simulink model "mysvm_svc"  (R2017b)
settings: Solver=ode45  StartTime=0.0  StopTime=0.02  RelTol=1e-3  EnableMultiTasking=on
values from neighbouring files (symbols this model uses):
  N = nlcinput(4) - 1    [MLNLC_m.m]    (also in MLPDPWM_m.m = pdpwminput(4) - 1; MLSVC_m.m = svcinput(4) - 1; MLSVM_m_HD.m = svminput(5) - 1; PlotSpaceVector.m = block.DialogPrm(1).Data - 1)
undefined symbols (not defined in the file or in its folder): m
libraries: powerlib x5, powerlib_meascontrol x5
settings Model: Creator=吴鸿达  LastModifiedBy=AdamWu
settings DataIOCC: LimitDataPoints=on  SaveFormat=Array
settings OptimizationCC: LifeSpan=inf
settings DebuggingCC: SolverPrmCheckMsg=warning  SFUnexpectedBacktrackingDiag=warning  SFNoUnconditionalDefaultTransitionDiag=warning  SFExecutionAtInitializationDiag=none
settings HardwareCC: ProdBitPerPointer=32  ProdBitPerSizeT=32  ProdBitPerPtrDiffT=32  ProdLargestAtomicFloat=None  ProdIntDivRoundTo=Undefined  ProdEndianess=Unspecified  ProdWordSize=32  ProdHWDeviceType=32-bit Generic
settings ModelReferenceCC: PropagateSignalLabelsOutOfModel=off
settings CodeAppCC: StateflowObjectComments=on
settings GRTTargetCC: TargetLangStandard=C89/C90 (ANSI)  GeneratePreprocessorConditionals=Disable all
settings ConfigComp: CovMetricSettings=dw  CovHtmlReporting=on  CovSaveCumulativeToWorkspaceVar=on  CovSaveSingleToWorkspaceVar=on  CovExternalEMLEnable=off  CovSFcnEnable=off
settings SimscapeCC: SimscapeNormalizeSystem=off

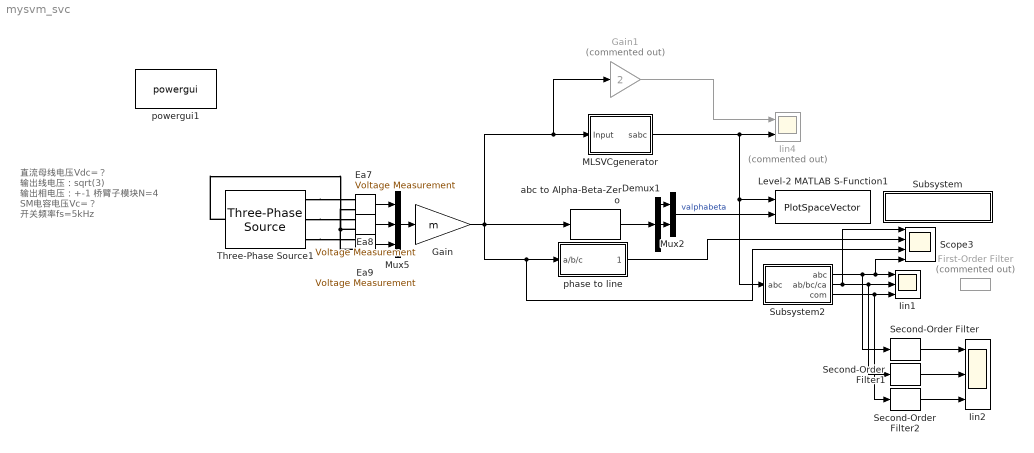
== system mysvm_svc ==
  note: 直流母线电压Vdc=？
      |
      | 输出线电压：sqrt(3)
      | 输出相电压：+-1
      | 桥臂子模块N=4
      | SM电容电压Vc=？
      | 开关频率fs=5kHz
  Demux1 : Demux  Outputs=3
  Ea7 : powerlib/Measurements/Voltage Measurement  PhasorSimulation=off  OutputType=Complex  PSBequivalent=0
  Ea8 : powerlib/Measurements/Voltage Measurement  PhasorSimulation=off  OutputType=Complex  PSBequivalent=0
  Ea9 : powerlib/Measurements/Voltage Measurement  PhasorSimulation=off  OutputType=Complex  PSBequivalent=0
  First-Order Filter : powerlib_meascontrol/Filters/First-Order Filter  Commented=on  FilterType=Lowpass  Tc=3.7e-4  Ts=0  Initialize=on  Vac_Init=[0, 0, 50]  Vdc_Init=0  PlotResponse=off  FreqRange="[0,  2000,  1]"
      settings: SourceProductName=Simscape Power Systems
  Gain : Gain  Gain=m
  Gain1 : Gain  Commented=on  Gain=2
  Iin1 : Scope  NumInputPorts=3
  Iin2 : Scope  NumInputPorts=3
  Iin4 : Scope  Commented=on  NumInputPorts=2
  Level-2 MATLAB S-Function1 : M-S-Function  FunctionName=PlotSpaceVector  Parameters=level, vdc, rate, normalized, plot, hexagon, sw, disabled  mask{disabled=off, level=N, rate=100, vdc=2/50, normalized=on, plot=5, hexagon=off, sw=off}
      mask prompts: disabled "Disable Plot"; level "Voltage Level"; rate "Plot Rate"; vdc "DC Link Voltage"; plot "Plot Number"; sw "Show Switching"
  MLSVCgenerator : Subsystem  mask{level=N, method=15. Zero Common Voltage}
      mask prompts: level "Voltage Level"
      mask TypeOptions method: 1. Conventional (x-y) | 2. x-y (iterative) | 3. H-D | 4. H-D (iterative) | 5. B-J-120 | 6. B-J-120 (iterative) | 7. B-J-60 | 8. B-J-60 (iterative) | 9. A-B-C | 10. A-B-C (iterative) | 11. Six-Axes | 12. Six-Axes (iterative) | 13. Shifted H-D | 14. Shifted B-J-60 | 15. Zero Common Voltage
  Mux2 : Mux  Inputs=2
  Mux5 : Mux  Inputs=3
  Scope3 : Scope  NumInputPorts=4
  Second-Order Filter : powerlib_meascontrol/Filters/Second-Order Filter  FilterType=Lowpass  Fo=1000  Zeta=0.707  Ts=0  Initialize=on  Vac_Init="[0,  0,  50]"  Vdc_Init=0  PlotResponse=off  FreqRange=[0, 500, 1]
      settings: SourceProductName=Simscape Power Systems  SourceProductBaseCode=PS
  Second-Order Filter1 : powerlib_meascontrol/Filters/Second-Order Filter  FilterType=Lowpass  Fo=1000  Zeta=0.707  Ts=0  Initialize=on  Vac_Init="[0,  0,  50]"  Vdc_Init=0.5  PlotResponse=off  FreqRange=[0, 500, 1]
      settings: SourceProductName=Simscape Power Systems  SourceProductBaseCode=PS
  Second-Order Filter2 : powerlib_meascontrol/Filters/Second-Order Filter  FilterType=Lowpass  Fo=1000  Zeta=0.707  Ts=0  Initialize=on  Vac_Init="[0,  0,  50]"  Vdc_Init=0.5  PlotResponse=off  FreqRange=[0, 500, 1]
      settings: SourceProductName=Simscape Power Systems  SourceProductBaseCode=PS
  Subsystem : Subsystem  mask{filename=SVPWM_sFunction.m}
      settings: AttributesFormatString=\n  OpenFcn=open('F:\研究生\matlab\PlotSpaceVector.m')
      mask Display:
      | patch([0 1 1 0], [0 0 1 1],[0.2 0.6 0.9])
      | disp('plotspacevector.m')
  Subsystem2 : Subsystem  mask{N=N, normal=on}
      mask prompts: N "Voltage Level"; normal "Normalized"
  Three-Phase Source1 : powerlib/Electrical Sources/Three-Phase Source  InternalConnection=Yn  VoltagePhases=off  Voltage=sqrt(2)  PhaseAngle=0  Voltage_phases=[25e3 25e3 25e3]/sqrt(3)  PhaseAngles_phases=[0 -120 +120]  Frequency=50  NonIdealSource=off  SpecifyImpedance=off  Resistance=0.8929  Inductance=1e-3  ShortCircuitLevel=100e6  BaseVoltage=25e3  XRratio=7  BusType=swing  Pref=10e3  Qref=0  Prefabc=[10e3, 10e3, 10e3]  Qrefabc=[0, 0, 0]  Qmin=-inf  Qmax=inf
  abc to Alpha-Beta-Zero : powerlib_meascontrol/Transformations/abc to Alpha-Beta-Zero
      settings: SourceProductName=Simscape Power Systems
  phase to line : Subsystem
  powergui1 : powerlib/powergui  Priority=1  SimulationMode=Discrete  SampleTime=0.5e-6  frequency=60  Iterations=50  frequencyindice=50  Pbase=100e6  ErrMax=1e-4  UnitsV=kV  UnitsW=MW  buscounter=0  FunctionMessages=off  echomessages=off  EnableUseOfTLC=off  CurrentSourceSwitches=off  DisableSnubberDevices=off  DisableRonSwitches=off  DisableVfSwitches=off  DisplayEquations=off  SolverType=Tustin/Backward Euler (TBE)  Interpol=off  ExternalGateDelay=off  methode=off  Ts=100  x0status=blocks  SPID=on  SwTol=0  HookPort=off  RestoreLinks=warning  ResistiveCurrentMeasurement=off  Frange=[0:2:500]  Ylog=off  Xlog=on  ShowGrid=off  save=off  variable=ZData  structure=SVMoutput  ZoomFFT=off  StartTime=0.00  cycles=1  DisplayStyle=3  fundamental=50  FreqAxis=on  MaxFrequency=15000  frequencyindicesteady=1  RmsSteady=1  display=off
  wires:
  Ea9/1 -> Mux5/3
  Ea7/1 -> Mux5/1
  Ea8/1 -> Mux5/2
  abc to Alpha-Beta-Zero/1 -> Demux1/1
  Demux1/1 -> Mux2/1
  Demux1/2 -> Mux2/2
  Mux5/1 -> Gain/1
  Mux2/1 -> Level-2 MATLAB S-Function1/2  "valphabeta"
  Subsystem2/2(ab/bc/ca) -> Scope3/1, Second-Order Filter1/1, Iin1/2
  Subsystem2/3(com) -> Second-Order Filter2/1, Iin1/3
  Subsystem2/1(abc) -> Second-Order Filter/1, Scope3/4, Iin1/1
  MLSVCgenerator/1(sabc) -> Subsystem2/1("abc "), Level-2 MATLAB S-Function1/1, Iin4/2
  Gain/1 -> Scope3/3, phase to line/1(a/b/c), Gain1/1, MLSVCgenerator/1(Input), abc to Alpha-Beta-Zero/1
  Gain1/1 -> Iin4/1
  Second-Order Filter/1 -> Iin2/1
  Second-Order Filter1/1 -> Iin2/2
  Second-Order Filter2/1 -> Iin2/3
  phase to line/1(ab/bc/ca) -> Scope3/2
  connections:
  Ea9/LConn2 -- Three-Phase Source1/LConn1 -- Ea7/LConn2 -- Ea8/LConn2
  Three-Phase Source1/RConn1 -- Ea7/LConn1
  Three-Phase Source1/RConn2 -- Ea8/LConn1
  Three-Phase Source1/RConn3 -- Ea9/LConn1

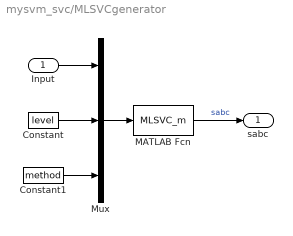
== system mysvm_svc/MLSVCgenerator ==
  Input : Inport
  Constant : Constant  Value=level
  Constant1 : Constant  Value=method
  MATLAB Fcn : MATLABFcn  MATLABFcn=MLSVC_m  OutputSignalType=real
  Mux : Mux  Inputs=3
  sabc : Outport
  wires:
  MATLAB Fcn/1 -> sabc/1  "sabc"
  Input/1 -> Mux/1
  Constant/1 -> Mux/2
  Mux/1 -> MATLAB Fcn/1
  Constant1/1 -> Mux/3

== system mysvm_svc/Subsystem ==

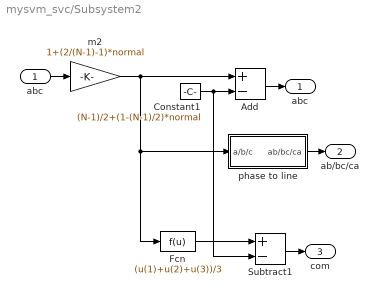
== system mysvm_svc/Subsystem2 ==
  "abc " : Inport
  Add : Sum  Inputs=+-
  Constant1 : Constant  Value=(N-1)/2+(1-(N-1)/2)*normal
  Fcn : Fcn  Expr=(u(1)+u(2)+u(3))/3
  Subtract1 : Sum  Inputs=+-
  m2 : Gain  Gain=1+(2/(N-1)-1)*normal
  phase to line : Subsystem
  abc : Outport
  ab/bc/ca : Outport  Port=2
  com : Outport  Port=3
  wires:
  Subtract1/1 -> com/1
  "abc "/1 -> m2/1
  Fcn/1 -> Subtract1/1
  Constant1/1 -> Subtract1/2, Add/2
  m2/1 -> Add/1, phase to line/1(a/b/c), Fcn/1
  Add/1 -> abc/1
  phase to line/1(ab/bc/ca) -> ab/bc/ca/1

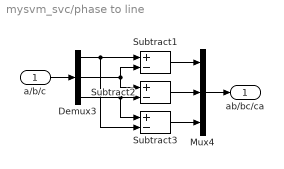
== system mysvm_svc/phase to line ==
  a/b/c : Inport
  Demux3 : Demux  Outputs=3
  Mux4 : Mux  Inputs=3
  Subtract1 : Sum  Inputs=+-
  Subtract2 : Sum  Inputs=+-
  Subtract3 : Sum  Inputs=+-
  ab/bc/ca : Outport
  wires:
  Subtract2/1 -> Mux4/2
  Subtract1/1 -> Mux4/1
  Demux3/2 -> Subtract2/1, Subtract1/2
  a/b/c/1 -> Demux3/1
  Mux4/1 -> ab/bc/ca/1
  Demux3/3 -> Subtract2/2, Subtract3/1
  Subtract3/1 -> Mux4/3
  Demux3/1 -> Subtract1/1, Subtract3/2

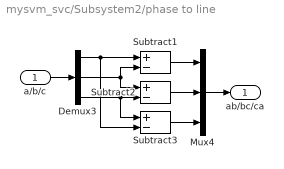
== system mysvm_svc/Subsystem2/phase to line ==
  a/b/c : Inport
  Demux3 : Demux  Outputs=3
  Mux4 : Mux  Inputs=3
  Subtract1 : Sum  Inputs=+-
  Subtract2 : Sum  Inputs=+-
  Subtract3 : Sum  Inputs=+-
  ab/bc/ca : Outport
  wires:
  Subtract2/1 -> Mux4/2
  Subtract1/1 -> Mux4/1
  Demux3/2 -> Subtract2/1, Subtract1/2
  a/b/c/1 -> Demux3/1
  Mux4/1 -> ab/bc/ca/1
  Demux3/3 -> Subtract2/2, Subtract3/1
  Subtract3/1 -> Mux4/3
  Demux3/1 -> Subtract1/1, Subtract3/2
